simulink model "parallhla"  (R2021a)
settings: Solver=ode23tb  StartTime=0.0  StopTime=45  MaxStep=1e-4  RelTol=1e-3
libraries: spsSeriesRLCBranchLib x7, spsCurrentMeasurementLib x4, simulink x4, spsDCMachineLib x2, spsDCVoltageSourceLib x2, spsControlledCurrentSourceLib x2, spsVoltageMeasurementLib x2, spsGroundLib x1, spspowerguiLib x1
settings Model: Creator=sotos  LastModifiedBy=sotos

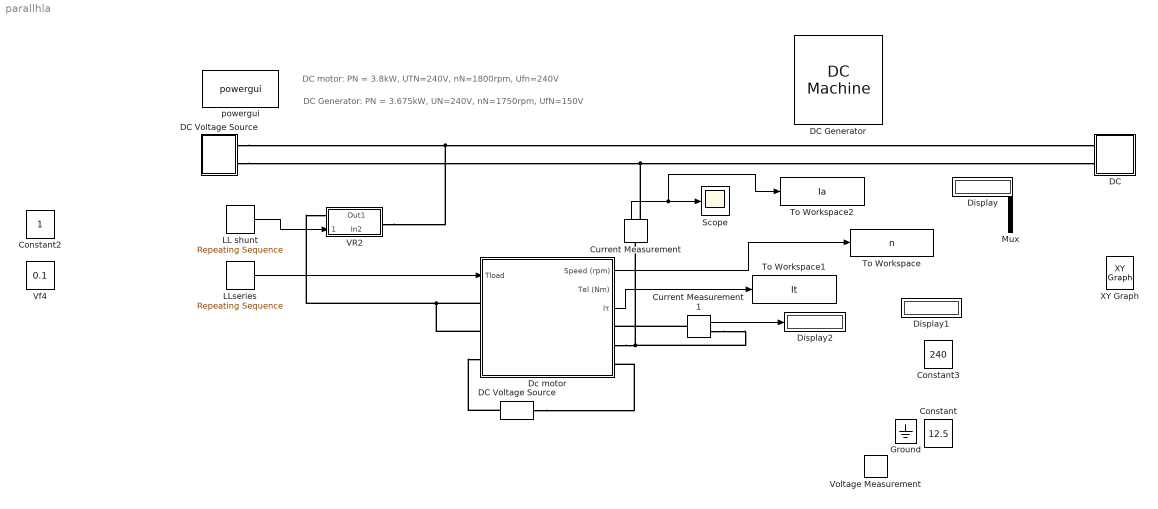
== system parallhla ==
  note: DC motor: PN = 3.8kW, UTN=240V, nN=1800rpm, Ufn=240V
  note: DC Generator: PN = 3.675kW, UN=240V, nN=1750rpm, UfN=150V
  Constant : Constant  Value=12.5
  Constant2 : Constant
  Constant3 : Constant  Value=240
  Current Measurement : spsCurrentMeasurementLib/Current Measurement  PhasorSimulation=off  OutputType=Complex  PSBequivalent=0
  Current Measurement1 : spsCurrentMeasurementLib/Current Measurement  PhasorSimulation=off  OutputType=Complex  PSBequivalent=0
  DC : Subsystem
  DC Generator : spsDCMachineLib/DC Machine  PresetModel=02: 5HP 240V 1750RPM Field:150V  MechanicalLoad=Torque TL  FieldType=Wound  ShowDetailedParameters=on  MeasurementBus=off  RLa=[0.78 0.016]  RLf=[150 112.5]  Laf=1.234  MachineConstant=Torque constant (N.m/A)  Ke=1.8  Kt=1.8  J=0.05  Bm=0.01  Tf=0  w0=1  Ifinit=1  TsPowergui=0  TsBlock=-1
  DC Voltage Source : Subsystem
  DC Voltage Source : spsDCVoltageSourceLib/DC Voltage Source  Amplitude=0  Measurements=None
  Dc motor : Subsystem  mask{PN=3.8, VN=240, nN=1800}
      mask prompts: PN "PN (kW)"; VN "VN (V)"; nN "nN (rpm)"
      mask DialogControl Control2 Prompt: DC Motor
  Display : Display
  Display1 : Display
  Display2 : Display
  Ground : spsGroundLib/Ground  LConnTagsString=a
  LL shunt : simulink/Sources/Repeating Sequence  rep_seq_t=t  rep_seq_y=R
  LLseries : simulink/Sources/Repeating Sequence  rep_seq_t=t  rep_seq_y=M
  Mux : Mux  Inputs=2
  Scope : Scope
  To Workspace : ToWorkspace  VariableName=n  SaveFormat=Timeseries  SampleTime=-1
  To Workspace1 : ToWorkspace  VariableName=It  SaveFormat=Timeseries  SampleTime=-1
  To Workspace2 : ToWorkspace  VariableName=Ia  SaveFormat=Timeseries  SampleTime=-1
  VR2 : Subsystem
      settings: PortSchema="{\"entries\":[{\"content\":{\"sides\":[{\"content\":{\"connectorIds\":[\"In1\",\"LConn1\"]},\"type\":\"ConnectorPlacement.EquallySpacedRectSide\",\"uuid\":\"64fa341b-3ca0-47a6-81c0-86bb2fc53f2a\"},{\"content\":{\"connectorIds\":[\"RConn1\"],\"side\":\"RIGHT\"},\"type\":\"ConnectorPlacement.EquallySpacedRectSide\",\"uuid\":\"6185be9a-3140-4071-baee-b7da69dc3849\"},{\"content\":{\"connectorIds\":[\"In2\"],\"side\":\"TOP\"},\"type\":\"ConnectorPlacement.EquallySpacedRectSide\",\"uuid\":\"2d582ff6-db8c-4997-88b4-7240c31e0e06\"},{\"content\":{\"connectorIds\":[\"Out1\"],\"side\":\"BOTTOM\"},\"type\":\"ConnectorPlacement.EquallySpacedRectSide\",\"uuid\":\"cde6fa20-825b-4faf-b83e-712e9213b115\"}]},\"type\":\"ConnectorPlacement.EquallySpacedConnector\",\"uuid\":\"5c634fd4-254d-4d6d-b9ce-c608b6f44997\"}],\"packageUris\":[\"http://schema.mathworks.com/mf0/Connector/R2020b\"],\"version\":\"1.0\"}"
  Vf4 : simulink/Math Operations/Slider Gain  gain=0.1  low=0  high=240
  Voltage Measurement : spsVoltageMeasurementLib/Voltage Measurement  PhasorSimulation=off  OutputType=Complex  PSBequivalent=0
  XY Graph : simulink/Sinks/XY Graph  xmin=0  xmax=15  ymin=0  ymax=8000  st=-1
  powergui : spspowerguiLib/powergui  Priority=1  SimulationMode=Discrete  SampleTime=50e-6  frequency=60  Iterations=50  frequencyindice=0  Pbase=100e6  ErrMax=1e-4  UnitsV=kV  UnitsW=MW  buscounter=0  FunctionMessages=off  echomessages=off  EnableUseOfTLC=off  CurrentSourceSwitches=off  DisableSnubberDevices=off  DisableRonSwitches=off  DisableVfSwitches=off  DisplayEquations=off  AutomaticDiscreteSolvers=on  SolverType=Tustin/Backward Euler (TBE)  Interpol=off  ExternalGateDelay=off  methode=off  Ts=100  x0status=blocks  SPID=on  SwTol=0  HookPort=off  NonlinearTolerance=1e-4  nMaxIteration=100  ContinueOnMaxIteration=off  RestoreLinks=warning  ResistiveCurrentMeasurement=off  Frange=[0:2:500]  Ylog=off  Xlog=on  ShowGrid=off  save=off  variable=ZData  structure=0  ZoomFFT=off  StartTime=0.0  cycles=1  DisplayStyle=1  fundamental=60  FreqAxis=off  MaxFrequency=1000  frequencyindicesteady=1  RmsSteady=1  display=off
  wires:
  Dc motor/3(Ιτ) -> To Workspace1/1
  LL shunt/1 -> VR2/1(R_value)
  Current Measurement/1 -> To Workspace2/1, Scope/1
  Dc motor/1(Speed (rpm)) -> To Workspace/1
  LLseries/1 -> Dc motor/1(Tload)
  Current Measurement1/1 -> Display2/1
  connections:
  DC Voltage Source/RConn2 -- Current Measurement/RConn1 -- DC/LConn2
  DC Voltage Source/RConn1 -- DC/LConn1 -- VR2/RConn1
  Dc motor/RConn2 -- Current Measurement1/RConn1 -- Current Measurement/LConn1
  Dc motor/LConn1 -- Dc motor/LConn2 -- VR2/LConn1
  DC Voltage Source/LConn1 -- Dc motor/RConn3
  DC Voltage Source/RConn1 -- Dc motor/LConn3
  Current Measurement1/LConn1 -- Dc motor/RConn1

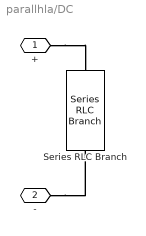
== system parallhla/DC ==
  Series RLC Branch : spsSeriesRLCBranchLib/Series RLC Branch  LConnTagsString=__new0  RConnTagsString=__new0  BranchType=R  Resistance=1e4  Inductance=1e-3  SetiL0=off  InitialCurrent=0  Capacitance=1e-6  Setx0=off  InitialVoltage=0  Measurements=None
  + : PMIOPort  Side=Left
  - : PMIOPort  Port=2  Side=Left
  connections:
  -/RConn1 -- Series RLC Branch/RConn1
  +/RConn1 -- Series RLC Branch/LConn1

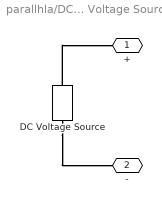
== system parallhla/DC Voltage Source ==
  DC Voltage Source : spsDCVoltageSourceLib/DC Voltage Source  Amplitude=240  Measurements=None
  + : PMIOPort  Side=Right
  - : PMIOPort  Port=2  Side=Right
  connections:
  DC Voltage Source/LConn1 -- -/RConn1
  DC Voltage Source/RConn1 -- +/RConn1

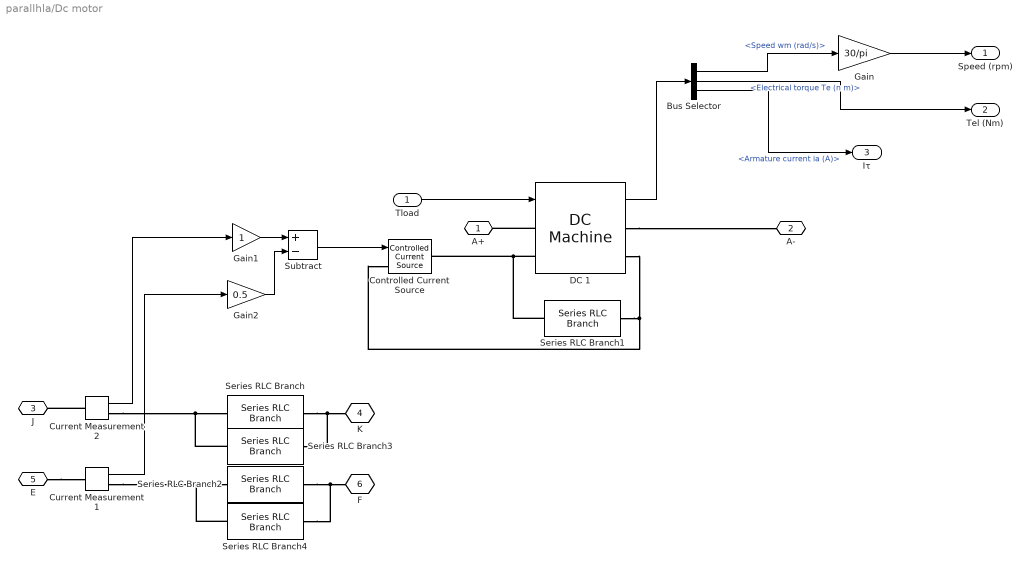
== system parallhla/Dc motor ==
  Tload : Inport
  Bus Selector : BusSelector  OutputSignals=Speed wm (rad/s),Electrical torque Te (n m),Armature current ia (A)
  Controlled Current Source : spsControlledCurrentSourceLib/Controlled Current Source  Initialize=on  Source_Type=DC  Amplitude=0  Phase=0  Frequency=0  Measurements=None
  Current Measurement1 : spsCurrentMeasurementLib/Current Measurement  PhasorSimulation=off  OutputType=Complex  PSBequivalent=0
  Current Measurement2 : spsCurrentMeasurementLib/Current Measurement  PhasorSimulation=off  OutputType=Complex  PSBequivalent=0
  DC 1 : spsDCMachineLib/DC Machine  PresetModel=No  MechanicalLoad=Torque TL  FieldType=Wound  ShowDetailedParameters=on  MeasurementBus=off  RLa=[0.78 0.016]  RLf=[150 60]  Laf=1.234  MachineConstant=Torque constant (N.m/A)  Ke=1.8  Kt=1.8  J=0.02  Bm=0.01  Tf=0  w0=0  Ifinit=0  TsPowergui=0  TsBlock=-1
  Gain : Gain  Gain=30/pi
  Gain1 : Gain
  Gain2 : Gain  Gain=0.5
  Series RLC Branch : spsSeriesRLCBranchLib/Series RLC Branch  LConnTagsString=__new0  RConnTagsString=__new0  BranchType=RL  Resistance=240  Inductance=120  SetiL0=off  InitialCurrent=0  Capacitance=1e-6  Setx0=off  InitialVoltage=0  Measurements=None
  Series RLC Branch1 : spsSeriesRLCBranchLib/Series RLC Branch  LConnTagsString=__new0  RConnTagsString=__new0  BranchType=R  Resistance=1e6  Inductance=120  SetiL0=off  InitialCurrent=0  Capacitance=1e-6  Setx0=off  InitialVoltage=0  Measurements=None
  Series RLC Branch2 : spsSeriesRLCBranchLib/Series RLC Branch  LConnTagsString=__new0  RConnTagsString=__new0  BranchType=RL  Resistance=0.1  Inductance=1e-3  SetiL0=off  InitialCurrent=0  Capacitance=1e-6  Setx0=off  InitialVoltage=0  Measurements=None
  Series RLC Branch3 : spsSeriesRLCBranchLib/Series RLC Branch  LConnTagsString=__new0  RConnTagsString=__new0  BranchType=R  Resistance=1e6  Inductance=120  SetiL0=off  InitialCurrent=0  Capacitance=1e-6  Setx0=off  InitialVoltage=0  Measurements=None
  Series RLC Branch4 : spsSeriesRLCBranchLib/Series RLC Branch  LConnTagsString=__new0  RConnTagsString=__new0  BranchType=R  Resistance=1e6  Inductance=120  SetiL0=off  InitialCurrent=0  Capacitance=1e-6  Setx0=off  InitialVoltage=0  Measurements=None
  Subtract : Sum  Inputs=+-
  A+ : PMIOPort  Side=Left
  A- : PMIOPort  Port=2  Side=Right
  J : PMIOPort  Port=3  Side=Left
  K : PMIOPort  Port=4  Side=Right
  E : PMIOPort  Port=5  Side=Left
  F : PMIOPort  Port=6  Side=Right
  Speed (rpm) : Outport
  Tel (Nm) : Outport  Port=2
  Ιτ : Outport  Port=3
  wires:
  Current Measurement2/1 -> Gain1/1
  Tload/1 -> DC 1/1
  Gain2/1 -> Subtract/2
  Current Measurement1/1 -> Gain2/1
  Subtract/1 -> Controlled Current Source/1
  Gain1/1 -> Subtract/1
  Bus Selector/2 -> Tel (Nm)/1  "<Electrical torque Te (n m)>"
  Gain/1 -> Speed (rpm)/1
  Bus Selector/1 -> Gain/1  "<Speed wm (rad/s)>"
  DC 1/1 -> Bus Selector/1
  Bus Selector/3 -> Ιτ/1  "<Armature current ia (A)>"
  connections:
  Series RLC Branch1/RConn1 -- DC 1/RConn2 -- Controlled Current Source/LConn1
  Series RLC Branch1/LConn1 -- DC 1/LConn2 -- Controlled Current Source/RConn1
  Current Measurement2/RConn1 -- Series RLC Branch3/LConn1 -- Series RLC Branch/LConn1
  DC 1/LConn1 -- A+/RConn1
  Current Measurement2/LConn1 -- J/RConn1
  DC 1/RConn1 -- A-/RConn1
  Series RLC Branch/RConn1 -- Series RLC Branch3/RConn1 -- K/RConn1
  E/RConn1 -- Current Measurement1/LConn1
  Current Measurement1/RConn1 -- Series RLC Branch4/LConn1 -- Series RLC Branch2/LConn1
  Series RLC Branch2/RConn1 -- Series RLC Branch4/RConn1 -- F/RConn1

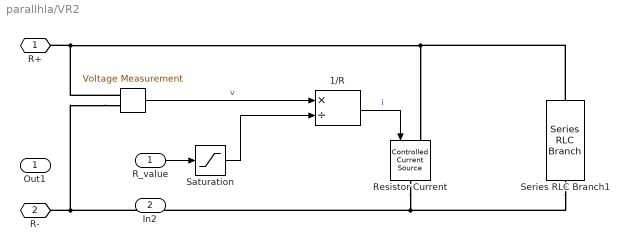
== system parallhla/VR2 ==
  R_value : Inport
  In2 : Inport  Port=2
  " " : spsVoltageMeasurementLib/Voltage Measurement  PhasorSimulation=off  OutputType=Magnitude  PSBequivalent=0
  1/R : Product  Inputs=*/  SaturateOnIntegerOverflow=on  OutDataTypeStr=Inherit: Same as first input
  Resistor Current : spsControlledCurrentSourceLib/Controlled Current Source  Initialize=off  Source_Type=DC  Amplitude=0  Phase=0  Frequency=0  Measurements=None
  Saturation : Saturate  UpperLimit=1e12  LowerLimit=0.01
  Series RLC Branch1 : spsSeriesRLCBranchLib/Series RLC Branch  LConnTagsString=__new0  RConnTagsString=__new0  BranchType=R  Resistance=1e6  Inductance=1e-3  SetiL0=off  InitialCurrent=0  Capacitance=1e-6  Setx0=off  InitialVoltage=0  Measurements=None
  R+ : PMIOPort  Side=Left
  R- : PMIOPort  Port=2  Side=Right
  Out1 : Outport
  wires:
  " "/1 -> 1/R/1  "v"
  1/R/1 -> Resistor Current/1  "i"
  R_value/1 -> Saturation/1
  Saturation/1 -> 1/R/2
  connections:
  " "/LConn1 -- Resistor Current/LConn1 -- Series RLC Branch1/LConn1 -- R+/RConn1
  " "/LConn2 -- Series RLC Branch1/RConn1 -- Resistor Current/RConn1 -- R-/RConn1
